simulink model "Autopilot_model"  (R2013a)
settings: Solver=ode45  StartTime=0.0  StopTime=10  FixedStep=.02  MaxStep=.02  RelTol=1e-3
model workspace (MAT data in the model file):
  op_trim1 : opcond.OperatingReport (value not decoded)
  op_snapshot1 : opcond.OperatingPoint (value not decoded)
values from neighbouring files (symbols this model uses):
  model = block.DialogPrm(1).Data    [copter_dynamics.m]
libraries: simulink x4
settings Model: Creator=Amir  LastModifiedBy=Amir
settings SolverCC: ZeroCrossAlgorithm=Adaptive  AutoInsertRateTranBlk=on
settings DataIOCC: ExternalInput=getinputstruct(op_snapshot1)  InitialState=getstatestruct(op_snapshot1)  LimitDataPoints=off  SignalLogging=off
settings DebuggingCC: MaxConsecutiveZCsMsg=none

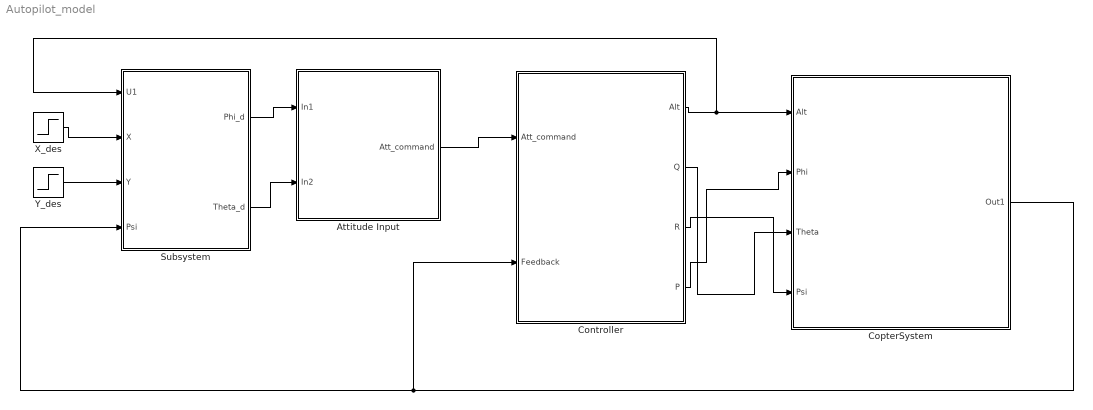
== system Autopilot_model ==
  Attitude Input : Subsystem
  Controller : Subsystem
  CopterSystem : Subsystem
  Subsystem : Subsystem
  X_des : Step  SampleTime=0
  Y_des : Step  Time=3  After=.5  SampleTime=0
  wires:
  Attitude Input/1(Att_command) -> Controller/1(Att_command)
  CopterSystem/1(Out1) -> Controller/2(Feedback), Subsystem/4(Psi)
  Controller/1("Alt ") -> Subsystem/1(U1), CopterSystem/1(Alt)
  Controller/3(R) -> CopterSystem/4(Psi)
  Controller/2(Q) -> CopterSystem/3(Theta)
  Controller/4("P ") -> CopterSystem/2(Phi)
  X_des/1 -> Subsystem/2(X)
  Y_des/1 -> Subsystem/3(Y)
  Subsystem/1(Phi_d) -> Attitude Input/1(In1)
  Subsystem/2(Theta_d) -> Attitude Input/2(In2)

== system Autopilot_model/Attitude Input ==
  In1 : Inport
  In2 : Inport  Port=2
  Bus Creator : BusCreator
  Step : Step  Time=0  Before=2  After=2.5  SampleTime=0
  Step1 : Step  Time=0  After=0  SampleTime=0
  Att_command : Outport
  wires:
  Bus Creator/1 -> Att_command/1
  Step1/1 -> Bus Creator/4  "Psi"
  In1/1 -> Bus Creator/2  "Phi"
  In2/1 -> Bus Creator/3  "Theta"
  Step/1 -> Bus Creator/1  "Alt"

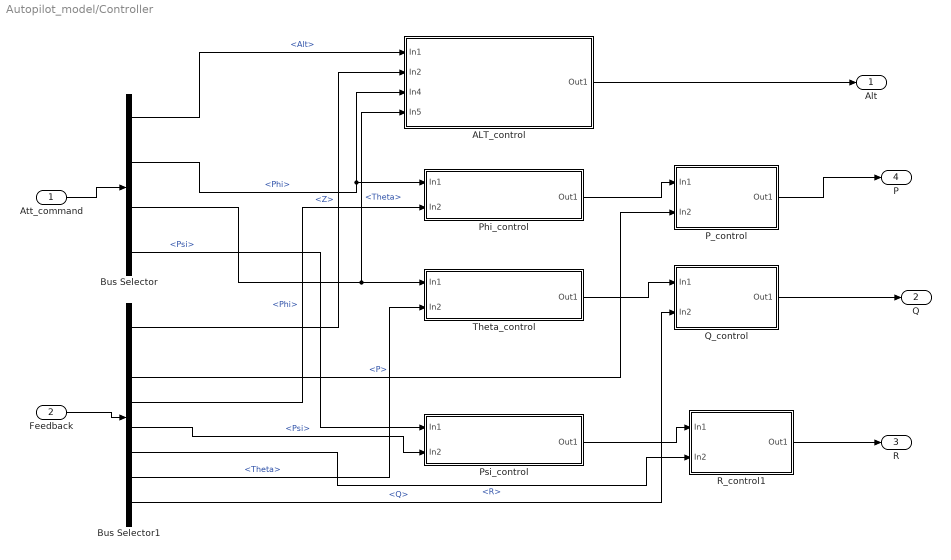
== system Autopilot_model/Controller ==
  Att_command : Inport
  Feedback : Inport  Port=2
  ALT_control : Subsystem
  Bus Selector : BusSelector  OutputSignals=Alt,Phi,Theta,Psi
  Bus Selector1 : BusSelector  OutputSignals=Z,W,P,Phi,Psi,R,Theta,Q
  P_control : Subsystem
  Phi_control : Subsystem
  Psi_control : Subsystem
  Q_control : Subsystem
  R_control1 : Subsystem
  Theta_control : Subsystem
  "Alt " : Outport
  Q : Outport  Port=2
  R : Outport  Port=3
  "P " : Outport  Port=4
  wires:
  Feedback/1 -> Bus Selector1/1
  Att_command/1 -> Bus Selector/1
  Bus Selector1/1 -> ALT_control/2(In2)  "<Z>"
  Bus Selector1/6 -> R_control1/2(In2)  "<R>"
  Bus Selector1/5 -> Psi_control/2(In2)  "<Psi>"
  Bus Selector/2 -> ALT_control/3(In4), Phi_control/1(In1)  "<Phi>"
  Bus Selector1/4 -> Phi_control/2(In2)  "<Phi>"
  Phi_control/1(Out1) -> P_control/1(In1)
  Bus Selector/3 -> Theta_control/1(In1), ALT_control/4(In5)  "<Theta>"
  Bus Selector1/7 -> Theta_control/2(In2)  "<Theta>"
  Bus Selector1/8 -> Q_control/2(In2)  "<Q>"
  Bus Selector/1 -> ALT_control/1(In1)  "<Alt>"
  ALT_control/1(Out1) -> "Alt "/1
  P_control/1(Out1) -> "P "/1
  Bus Selector1/3 -> P_control/2(In2)  "<P>"
  Bus Selector/4 -> Psi_control/1(In1)  "<Psi>"
  Psi_control/1(Out1) -> R_control1/1(In1)
  R_control1/1(Out1) -> R/1
  Theta_control/1(Out1) -> Q_control/1(In1)
  Q_control/1(Out1) -> Q/1

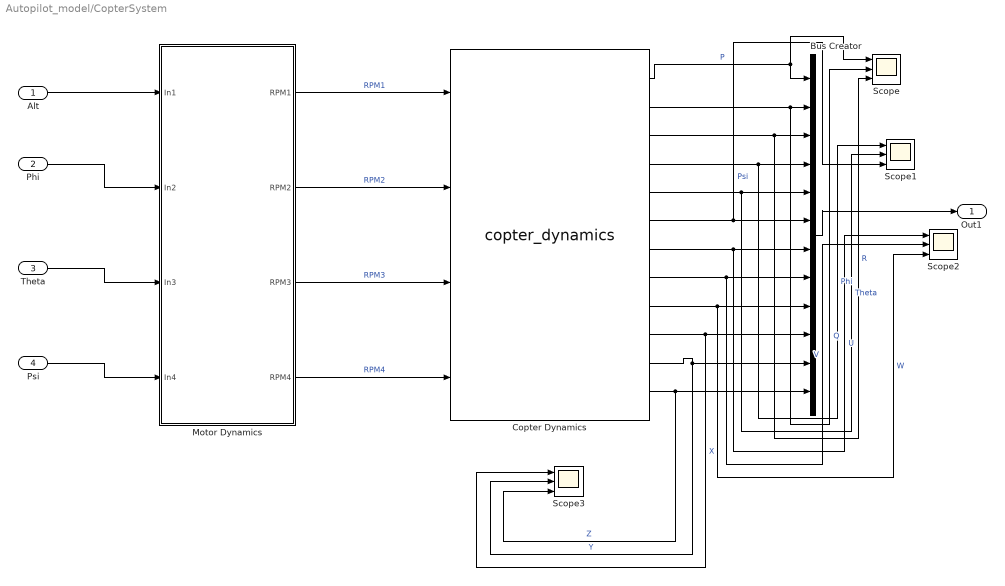
== system Autopilot_model/CopterSystem ==
  Alt : Inport
  Phi : Inport  Port=2
  Theta : Inport  Port=3
  Psi : Inport  Port=4
  Bus Creator : BusCreator  Inputs=12
  Copter Dynamics : M-S-Function  FunctionName=copter_dynamics  Parameters=model
  Motor Dynamics : Subsystem
  Scope{,1..3} (4 alike) : Scope  NumInputPorts=3
      Scope settings: YMin=-750~-750~-11050  YMax=750~750~-11010
      Scope1 settings: YMin=-0.06~-0.35~-0.027  YMax=0.07~0.35~-0.009
      Scope2 settings: YMin=-400~-350~2630  YMax=400~400~2700  SaveName=ScopeData2
      Scope3 settings: YMin=1.0018~7.3e-07~2.50025  YMax=1.0028~8.8e-07~2.50026  SaveName=ScopeData3
  Out1 : Outport
  wires:
  Alt/1 -> Motor Dynamics/1(In1)
  Copter Dynamics/9 -> Bus Creator/9, Scope2/3  "W"
  Copter Dynamics/3 -> Bus Creator/3, Scope/3  "R"
  Copter Dynamics/10 -> Bus Creator/10, Scope3/1  "X"
  Copter Dynamics/2 -> Bus Creator/2, Scope/2  "Q"
  Copter Dynamics/4 -> Bus Creator/4, Scope1/1  "Phi"
  Copter Dynamics/7 -> Bus Creator/7, Scope2/1  "U"
  Copter Dynamics/6 -> Bus Creator/6, Scope1/3  "Psi"
  Copter Dynamics/8 -> Bus Creator/8, Scope2/2  "V"
  Copter Dynamics/12 -> Bus Creator/12, Scope3/3  "Z"
  Copter Dynamics/5 -> Bus Creator/5, Scope1/2  "Theta"
  Bus Creator/1 -> Out1/1
  Copter Dynamics/11 -> Bus Creator/11, Scope3/2  "Y"
  Motor Dynamics/1(RPM1) -> Copter Dynamics/1  "RPM1"
  Motor Dynamics/2(RPM2) -> Copter Dynamics/2  "RPM2"
  Motor Dynamics/3(RPM3) -> Copter Dynamics/3  "RPM3"
  Motor Dynamics/4(RPM4) -> Copter Dynamics/4  "RPM4"
  Copter Dynamics/1 -> Scope/1, Bus Creator/1  "P"
  Psi/1 -> Motor Dynamics/4(In4)
  Theta/1 -> Motor Dynamics/3(In3)
  Phi/1 -> Motor Dynamics/2(In2)

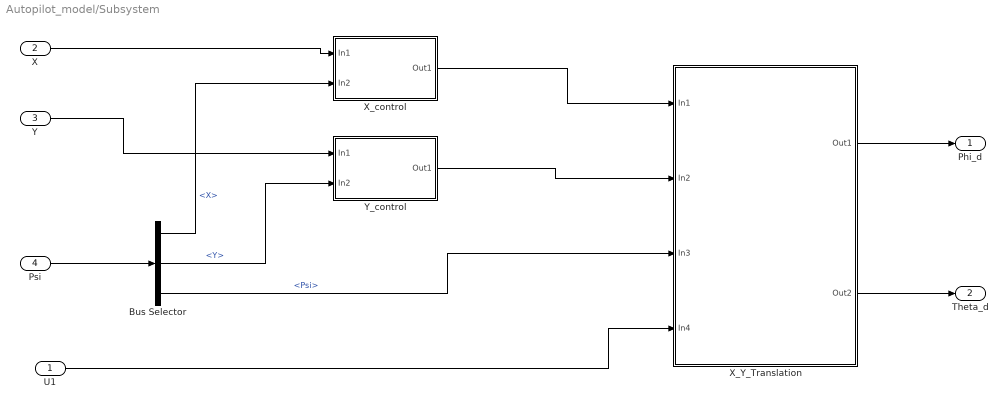
== system Autopilot_model/Subsystem ==
  U1 : Inport
  X : Inport  Port=2
  Y : Inport  Port=3
  Psi : Inport  Port=4
  Bus Selector : BusSelector  OutputSignals=X,Y,Psi
  X_Y_Translation : Subsystem
  X_control : Subsystem
  Y_control : Subsystem
  Phi_d : Outport
  Theta_d : Outport  Port=2
  wires:
  Psi/1 -> Bus Selector/1
  Bus Selector/3 -> X_Y_Translation/3(In3)  "<Psi>"
  X_Y_Translation/1(Out1) -> Phi_d/1
  X_Y_Translation/2(Out2) -> Theta_d/1
  X_control/1(Out1) -> X_Y_Translation/1(In1)
  Bus Selector/1 -> X_control/2(In2)  "<X>"
  X/1 -> X_control/1(In1)
  Y/1 -> Y_control/1(In1)
  Bus Selector/2 -> Y_control/2(In2)  "<Y>"
  U1/1 -> X_Y_Translation/4(In4)
  Y_control/1(Out1) -> X_Y_Translation/2(In2)

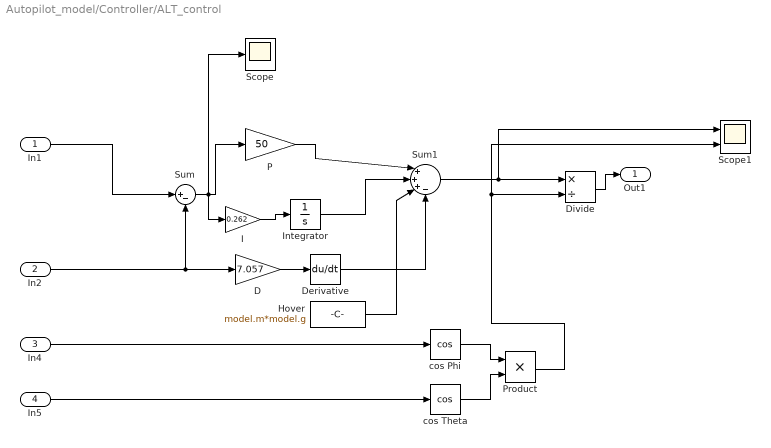
== system Autopilot_model/Controller/ALT_control ==
  In1 : Inport
  In2 : Inport  Port=2
  In4 : Inport  Port=3
  In5 : Inport  Port=4
  D : Gain  Gain=7.057
  Derivative : Derivative
  Divide : Product  Inputs=*/
  Hover : Constant  Value=model.m*model.g
  I : Gain  Gain=0.262
  Integrator : Integrator  LimitOutput=on  UpperSaturationLimit=1  LowerSaturationLimit=-1
  P : Gain  Gain=50
  Product : Product  RndMeth=Zero
  Scope : Scope
      settings: YMin=-0.1  YMax=1.2  SaveName=ScopeData6
  Scope1 : Scope  NumInputPorts=2
      settings: YMin=-0.1~-5  YMax=1.2~5  SaveName=ScopeData8
  Sum : Sum  Inputs=|+-
  Sum1 : Sum  Inputs=|+++-
  cos Phi : Trigonometry  Operator=cos
  cos Theta : Trigonometry  Operator=cos
  Out1 : Outport
  wires:
  In2/1 -> Sum/2, D/1
  P/1 -> Sum1/1
  In1/1 -> Sum/1
  Sum/1 -> Scope/1, I/1, P/1
  Integrator/1 -> Sum1/2
  I/1 -> Integrator/1
  Hover/1 -> Sum1/3
  cos Phi/1 -> Product/1
  cos Theta/1 -> Product/2
  In4/1 -> cos Phi/1
  In5/1 -> cos Theta/1
  Sum1/1 -> Scope1/1, Divide/1
  Divide/1 -> Out1/1
  Product/1 -> Scope1/2, Divide/2
  D/1 -> Derivative/1
  Derivative/1 -> Sum1/4

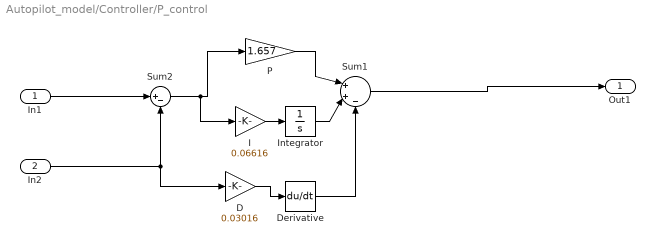
== system Autopilot_model/Controller/P_control ==
  In1 : Inport
  In2 : Inport  Port=2
  D : Gain  Gain=0.03016
  Derivative : Derivative
  I : Gain  Gain=0.06616
  Integrator : Integrator  LimitOutput=on  UpperSaturationLimit=1  LowerSaturationLimit=-1
  P : Gain  Gain=1.657
  Sum1 : Sum  Inputs=|++-
  Sum2 : Sum  Inputs=|+-
  Out1 : Outport
  wires:
  P/1 -> Sum1/1
  I/1 -> Integrator/1
  Sum1/1 -> Out1/1
  Integrator/1 -> Sum1/2
  In1/1 -> Sum2/1
  Sum2/1 -> I/1, P/1
  In2/1 -> Sum2/2, D/1
  Derivative/1 -> Sum1/3
  D/1 -> Derivative/1

== system Autopilot_model/Controller/Phi_control ==
  In1 : Inport
  In2 : Inport  Port=2
  P : Gain  Gain=6.22
  Sum : Sum  Inputs=|+-
  Out1 : Outport
  wires:
  Sum/1 -> P/1
  In1/1 -> Sum/1
  P/1 -> Out1/1
  In2/1 -> Sum/2

== system Autopilot_model/Controller/Psi_control ==
  In1 : Inport
  In2 : Inport  Port=2
  P : Gain  Gain=3
  Sum : Sum  Inputs=|+-
  Out1 : Outport
  wires:
  Sum/1 -> P/1
  In1/1 -> Sum/1
  P/1 -> Out1/1
  In2/1 -> Sum/2

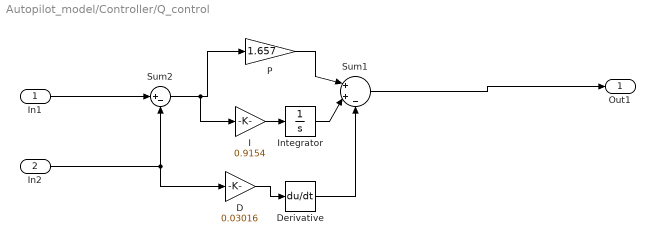
== system Autopilot_model/Controller/Q_control ==
  In1 : Inport
  In2 : Inport  Port=2
  D : Gain  Gain=0.03016
  Derivative : Derivative
  I : Gain  Gain=0.9154
  Integrator : Integrator  LimitOutput=on  UpperSaturationLimit=1  LowerSaturationLimit=-1
  P : Gain  Gain=1.657
  Sum1 : Sum  Inputs=|++-
  Sum2 : Sum  Inputs=|+-
  Out1 : Outport
  wires:
  P/1 -> Sum1/1
  I/1 -> Integrator/1
  Sum1/1 -> Out1/1
  Integrator/1 -> Sum1/2
  In1/1 -> Sum2/1
  Sum2/1 -> I/1, P/1
  In2/1 -> Sum2/2, D/1
  Derivative/1 -> Sum1/3
  D/1 -> Derivative/1

== system Autopilot_model/Controller/R_control1 ==
  In1 : Inport
  In2 : Inport  Port=2
  I : Gain  Gain=3.457
  Integrator : Integrator  LimitOutput=on  UpperSaturationLimit=1  LowerSaturationLimit=-1
  P : Gain  Gain=8.308
  Sum1 : Sum  Inputs=|++-
  Sum2 : Sum  Inputs=|+-
  Out1 : Outport
  wires:
  P/1 -> Sum1/1
  I/1 -> Integrator/1
  Sum1/1 -> Out1/1
  Integrator/1 -> Sum1/2
  In1/1 -> Sum2/1
  Sum2/1 -> I/1, P/1
  In2/1 -> Sum2/2

== system Autopilot_model/Controller/Theta_control ==
  In1 : Inport
  In2 : Inport  Port=2
  P : Gain  Gain=6.22
  Sum : Sum  Inputs=|+-
  Out1 : Outport
  wires:
  In2/1 -> Sum/2
  P/1 -> Out1/1
  In1/1 -> Sum/1
  Sum/1 -> P/1

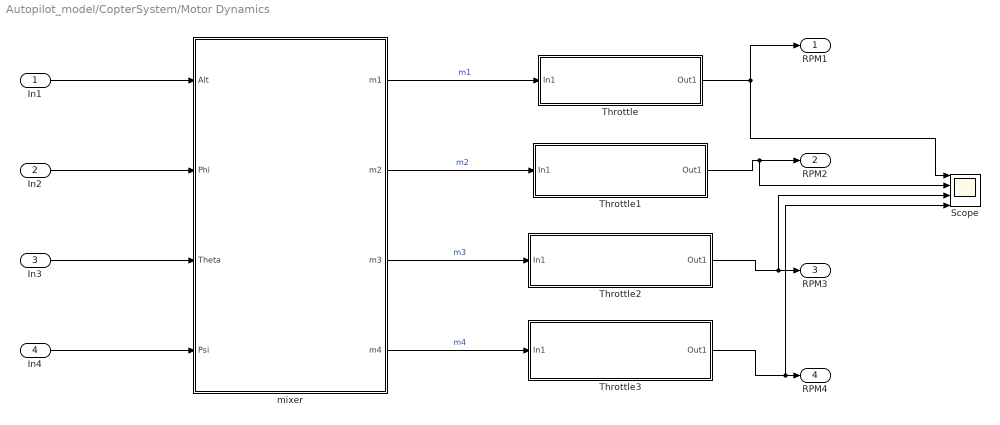
== system Autopilot_model/CopterSystem/Motor Dynamics ==
  In1 : Inport
  In2 : Inport  Port=2
  In3 : Inport  Port=3
  In4 : Inport  Port=4
  Scope : Scope  NumInputPorts=4
      settings: YMin=2500~2500~2500~2500  YMax=5250~5250~5250~5250  SaveName=ScopeData5
  Throttle : Subsystem
  Throttle1 : Subsystem
  Throttle2 : Subsystem
  Throttle3 : Subsystem
  mixer : Subsystem
  RPM1 : Outport
  RPM2 : Outport  Port=2
  RPM3 : Outport  Port=3
  RPM4 : Outport  Port=4
  wires:
  Throttle/1(Out1) -> RPM1/1, Scope/1
  Throttle2/1(Out1) -> Scope/3, RPM3/1
  Throttle3/1(Out1) -> Scope/4, RPM4/1
  In1/1 -> mixer/1(Alt)
  In2/1 -> mixer/2(Phi)
  In3/1 -> mixer/3(Theta)
  In4/1 -> mixer/4(Psi)
  mixer/1(m1) -> Throttle/1(In1)  "m1"
  mixer/2(m2) -> Throttle1/1(In1)  "m2"
  mixer/3(m3) -> Throttle2/1(In1)  "m3"
  mixer/4(m4) -> Throttle3/1(In1)  "m4"
  Throttle1/1(Out1) -> Scope/2, RPM2/1

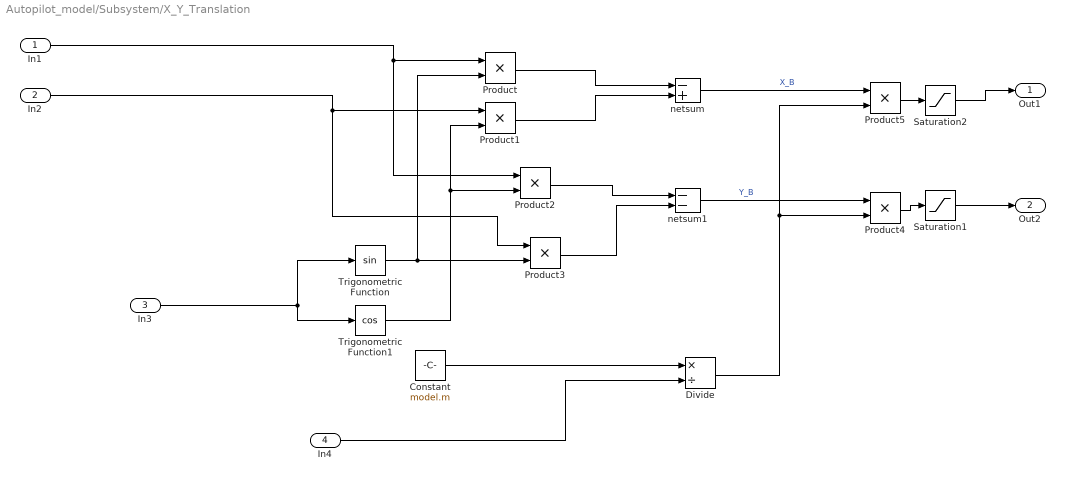
== system Autopilot_model/Subsystem/X_Y_Translation ==
  In1 : Inport
  In2 : Inport  Port=2
  In3 : Inport  Port=3
  In4 : Inport  Port=4
  Constant : Constant  Value=model.m
  Divide : Product  Inputs=*/
  Product{,1..5} (6 alike) : Product
  Saturation1 : Saturate  UpperLimit=30*pi/180  LowerLimit=-30*pi/180
  Saturation2 : Saturate  UpperLimit=30*pi/180  LowerLimit=-30*pi/180
  Trigonometric Function : Trigonometry
  Trigonometric Function1 : Trigonometry  Operator=cos
  netsum : Sum  Inputs=-+  SaturateOnIntegerOverflow=on  InputSameDT=on  OutDataTypeStr=Inherit: Same as first input
  netsum1 : Sum  Inputs=--  SaturateOnIntegerOverflow=on  InputSameDT=on  OutDataTypeStr=Inherit: Same as first input
  Out1 : Outport
  Out2 : Outport  Port=2
  wires:
  Divide/1 -> Product4/2, Product5/2
  netsum/1 -> Product5/1  "X_B"
  netsum1/1 -> Product4/1  "Y_B"
  Product/1 -> netsum/1
  In3/1 -> Trigonometric Function1/1, Trigonometric Function/1
  In1/1 -> Product2/1, Product/1
  Trigonometric Function/1 -> Product/2, Product3/2
  Product1/1 -> netsum/2
  In2/1 -> Product3/1, Product1/1
  Product2/1 -> netsum1/1
  Trigonometric Function1/1 -> Product2/2, Product1/2
  Product3/1 -> netsum1/2
  Constant/1 -> Divide/1
  Saturation1/1 -> Out2/1
  Saturation2/1 -> Out1/1
  In4/1 -> Divide/2
  Product5/1 -> Saturation2/1
  Product4/1 -> Saturation1/1

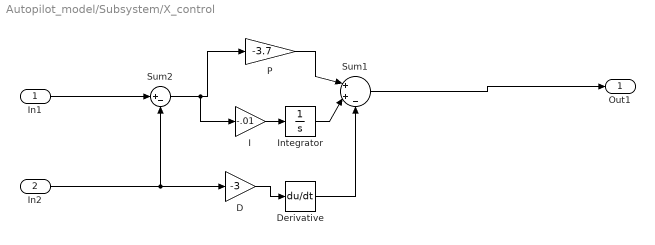
== system Autopilot_model/Subsystem/X_control ==
  In1 : Inport
  In2 : Inport  Port=2
  D : Gain  Gain=-3
  Derivative : Derivative
  I : Gain  Gain=-.01
  Integrator : Integrator  LimitOutput=on  UpperSaturationLimit=1  LowerSaturationLimit=-1
  P : Gain  Gain=-3.7
  Sum1 : Sum  Inputs=|++-
  Sum2 : Sum  Inputs=|+-
  Out1 : Outport
  wires:
  P/1 -> Sum1/1
  I/1 -> Integrator/1
  Sum1/1 -> Out1/1
  Integrator/1 -> Sum1/2
  In1/1 -> Sum2/1
  Sum2/1 -> I/1, P/1
  In2/1 -> Sum2/2, D/1
  Derivative/1 -> Sum1/3
  D/1 -> Derivative/1

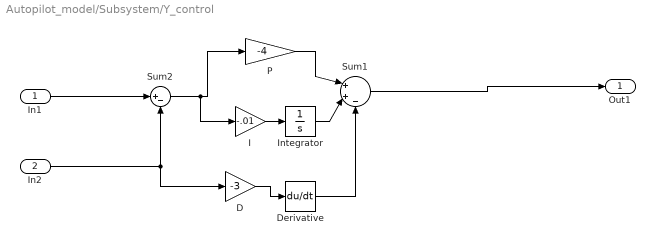
== system Autopilot_model/Subsystem/Y_control ==
  In1 : Inport
  In2 : Inport  Port=2
  D : Gain  Gain=-3
  Derivative : Derivative
  I : Gain  Gain=-.01
  Integrator : Integrator  LimitOutput=on  UpperSaturationLimit=1  LowerSaturationLimit=-1
  P : Gain  Gain=-4
  Sum1 : Sum  Inputs=|++-
  Sum2 : Sum  Inputs=|+-
  Out1 : Outport
  wires:
  D/1 -> Derivative/1
  Derivative/1 -> Sum1/3
  In2/1 -> D/1, Sum2/2
  Sum2/1 -> P/1, I/1
  In1/1 -> Sum2/1
  Integrator/1 -> Sum1/2
  Sum1/1 -> Out1/1
  I/1 -> Integrator/1
  P/1 -> Sum1/1

== system Autopilot_model/CopterSystem/Motor Dynamics/Throttle ==
  In1 : Inport
  Compare To Constant : simulink/Logic and Bit Operations/Compare To Constant  relop=>=  const=model.minThrottle  OutDataTypeStr=uint8  ZeroCross=off
  Constant : Constant  Value=model.K
  Gain : Gain  Gain=model.C
  Product : Product
  Saturation : Saturate  UpperLimit=40  LowerLimit=0
  Sum : Sum  Inputs=|++
  Out1 : Outport
  wires:
  In1/1 -> Compare To Constant/1, Saturation/1
  Gain/1 -> Sum/1
  Constant/1 -> Sum/2
  Saturation/1 -> Gain/1
  Sum/1 -> Product/1
  Product/1 -> Out1/1
  Compare To Constant/1 -> Product/2

== system Autopilot_model/CopterSystem/Motor Dynamics/Throttle1 ==
  In1 : Inport
  Compare To Constant : simulink/Logic and Bit Operations/Compare To Constant  relop=>=  const=model.minThrottle  OutDataTypeStr=uint8  ZeroCross=off
  Constant1 : Constant  Value=model.K
  Gain1 : Gain  Gain=model.C
  Product : Product
  Saturation1 : Saturate  UpperLimit=40  LowerLimit=0
  Sum1 : Sum  Inputs=|++
  Out1 : Outport
  wires:
  In1/1 -> Compare To Constant/1, Saturation1/1
  Gain1/1 -> Sum1/1
  Constant1/1 -> Sum1/2
  Saturation1/1 -> Gain1/1
  Sum1/1 -> Product/1
  Product/1 -> Out1/1
  Compare To Constant/1 -> Product/2

== system Autopilot_model/CopterSystem/Motor Dynamics/Throttle2 ==
  In1 : Inport
  Compare To Constant : simulink/Logic and Bit Operations/Compare To Constant  relop=>=  const=model.minThrottle  OutDataTypeStr=uint8  ZeroCross=off
  Constant : Constant  Value=model.K
  Gain : Gain  Gain=model.C
  Product : Product
  Saturation : Saturate  UpperLimit=40  LowerLimit=0
  Sum : Sum  Inputs=|++
  Out1 : Outport
  wires:
  Gain/1 -> Sum/1
  Constant/1 -> Sum/2
  Saturation/1 -> Gain/1
  Sum/1 -> Product/1
  Product/1 -> Out1/1
  Compare To Constant/1 -> Product/2
  In1/1 -> Compare To Constant/1, Saturation/1

== system Autopilot_model/CopterSystem/Motor Dynamics/Throttle3 ==
  In1 : Inport
  Compare To Constant : simulink/Logic and Bit Operations/Compare To Constant  relop=>=  const=model.minThrottle  OutDataTypeStr=uint8  ZeroCross=off
  Constant : Constant  Value=model.K
  Gain : Gain  Gain=model.C
  Product : Product
  Saturation : Saturate  UpperLimit=40  LowerLimit=0
  Scope : Scope  NumInputPorts=2
      settings: YMin=-5~-5  YMax=5~5  SaveName=ScopeData4
  Sum : Sum  Inputs=|++
  Out1 : Outport
  wires:
  In1/1 -> Scope/2, Compare To Constant/1, Saturation/1
  Gain/1 -> Sum/1
  Constant/1 -> Sum/2
  Saturation/1 -> Gain/1
  Sum/1 -> Product/1
  Product/1 -> Out1/1
  Compare To Constant/1 -> Product/2, Scope/1

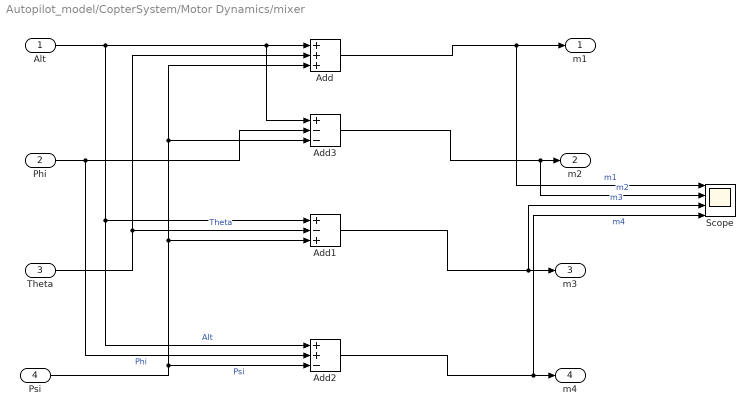
== system Autopilot_model/CopterSystem/Motor Dynamics/mixer ==
  Alt : Inport
  Phi : Inport  Port=2
  Theta : Inport  Port=3
  Psi : Inport  Port=4
  Add : Sum  Inputs=+++
  Add1 : Sum  Inputs=+-+
  Add2 : Sum  Inputs=++-
  Add3 : Sum  Inputs=+--
  Scope : Scope  NumInputPorts=4
      settings: YMin=-5~-5~-5~-5  YMax=5~5~5~5  SaveName=ScopeData9
  m1 : Outport
  m2 : Outport  Port=2
  m3 : Outport  Port=3
  m4 : Outport  Port=4
  wires:
  Alt/1 -> Add2/1, Add1/1, Add3/1, Add/1  "Alt"
  Psi/1 -> Add2/3, Add1/3, Add/3, Add3/3  "Psi"
  Theta/1 -> Add1/2, Add/2  "Theta"
  Phi/1 -> Add2/2, Add3/2  "Phi"
  Add2/1 -> Scope/4, m4/1  "m4"
  Add/1 -> Scope/1, m1/1  "m1"
  Add1/1 -> Scope/3, m3/1  "m3"
  Add3/1 -> Scope/2, m2/1  "m2"
